simulink model "Simulink_Modell_Aufgabe20"  (R2017b)
settings: Solver=VariableStepAuto  StartTime=0.0  StopTime=10.0  RelTol=1e-3
values from neighbouring files (symbols this model uses):
  A = double(vpa(A))    [Skript_Vorbereitung.m]
  Ar11 = Ar(1:n,1:n)    [Skript_Vorbereitung.m]
  Ar12 = Ar(1:n,n+1:length(A))    [Skript_Vorbereitung.m]
  Ar21 = Ar(n+1:length(A), 1:n)    [Skript_Vorbereitung.m]
  Ar22 = Ar(n+1:length(A),n+1:length(A))    [Skript_Vorbereitung.m]
  b = double(vpa(b))    [Skript_Vorbereitung.m]
  br1 = br(1:n)    [Skript_Vorbereitung.m]
  br2 = br(n+1:length(A))    [Skript_Vorbereitung.m]
  C = [1 0 0 0; 0 0 1 0]    [Skript_Vorbereitung.m]
  k = acker(A,b,p)    [Skript_Vorbereitung.m]
  L_red = L_riccati_red    [Skript_Vorbereitung.m]
settings Model: Creator=Lucas  LastModifiedBy=Lucas

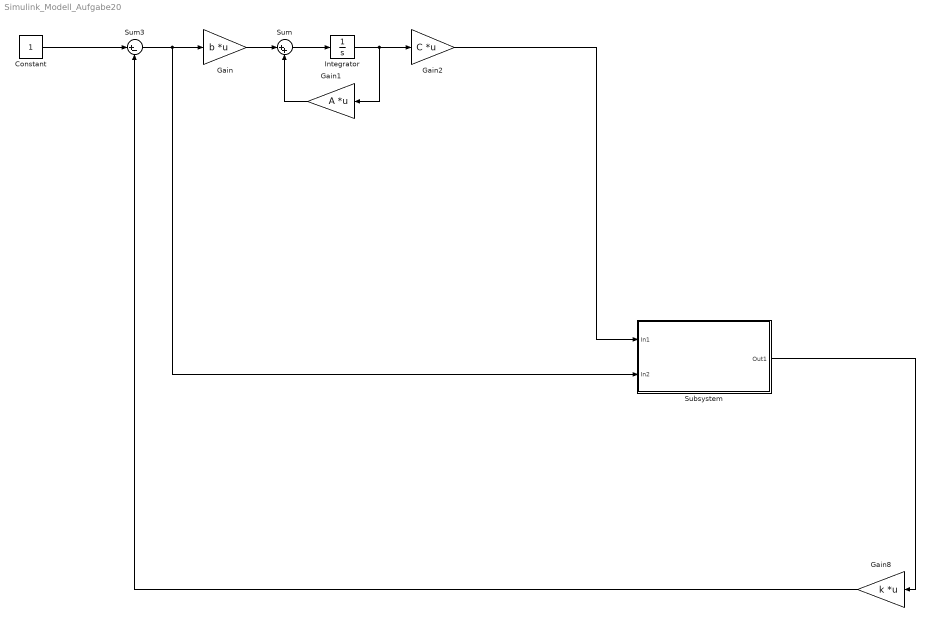
== system Simulink_Modell_Aufgabe20 ==
  Constant : Constant
  Gain : Gain  Gain=b  Multiplication=Matrix(K*u)
  Gain1 : Gain  Gain=A  Multiplication=Matrix(K*u)
  Gain2 : Gain  Gain=C  Multiplication=Matrix(K*u)
  Gain8 : Gain  Gain=k  Multiplication=Matrix(K*u)
  Integrator : Integrator
  Subsystem : Subsystem
  Sum : Sum  Inputs=|++
  Sum3 : Sum  Inputs=|+-
  wires:
  Sum/1 -> Integrator/1
  Gain/1 -> Sum/1
  Gain1/1 -> Sum/2
  Integrator/1 -> Gain2/1, Gain1/1
  Sum3/1 -> Subsystem/2(In2), Gain/1
  Constant/1 -> Sum3/1
  Gain8/1 -> Sum3/2
  Gain2/1 -> Subsystem/1(In1)
  Subsystem/1(Out1) -> Gain8/1

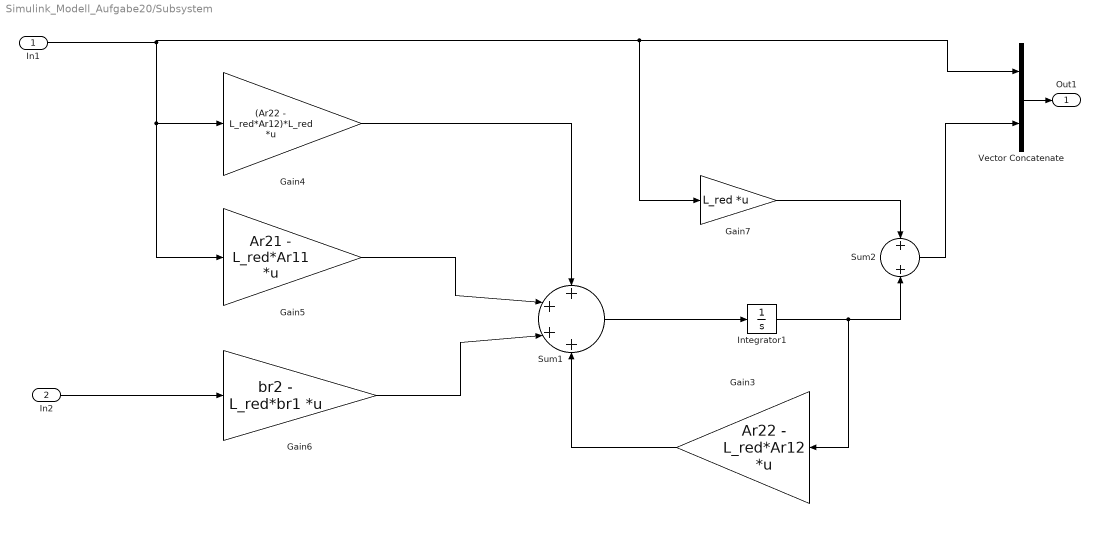
== system Simulink_Modell_Aufgabe20/Subsystem ==
  In1 : Inport
  In2 : Inport  Port=2
  Gain3 : Gain  Gain=Ar22 - L_red*Ar12  Multiplication=Matrix(K*u)
  Gain4 : Gain  Gain=(Ar22 - L_red*Ar12)*L_red  Multiplication=Matrix(K*u)
  Gain5 : Gain  Gain=Ar21 - L_red*Ar11  Multiplication=Matrix(K*u)
  Gain6 : Gain  Gain=br2 - L_red*br1  Multiplication=Matrix(K*u)
  Gain7 : Gain  Gain=L_red  Multiplication=Matrix(K*u)
  Integrator1 : Integrator
  Sum1 : Sum  Inputs=++++
  Sum2 : Sum
  Vector Concatenate : Concatenate
  Out1 : Outport
  wires:
  In2/1 -> Gain6/1
  Gain4/1 -> Sum1/1
  Vector Concatenate/1 -> Out1/1
  Gain3/1 -> Sum1/4
  Gain6/1 -> Sum1/3
  Sum2/1 -> Vector Concatenate/2
  In1/1 -> Vector Concatenate/1, Gain7/1, Gain5/1, Gain4/1
  Sum1/1 -> Integrator1/1
  Integrator1/1 -> Sum2/2, Gain3/1
  Gain5/1 -> Sum1/2
  Gain7/1 -> Sum2/1
